simulink model "task1"  (R2023b)
settings: Solver=VariableStepAuto  StartTime=0.0  StopTime=100  RelTol=1e-3
settings Model: Creator=Notebook  LastModifiedBy=Notebook

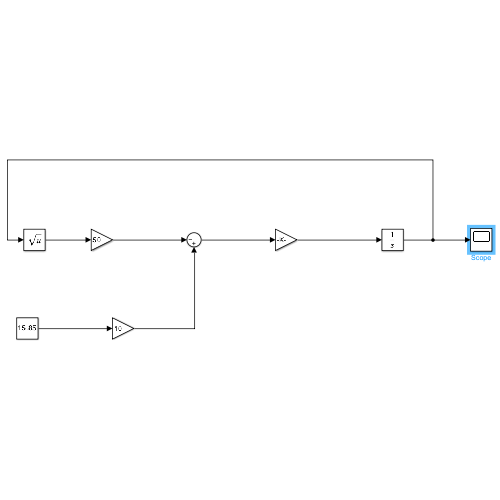
[thumbnail: Simulink's stored preview of the top-level diagram]
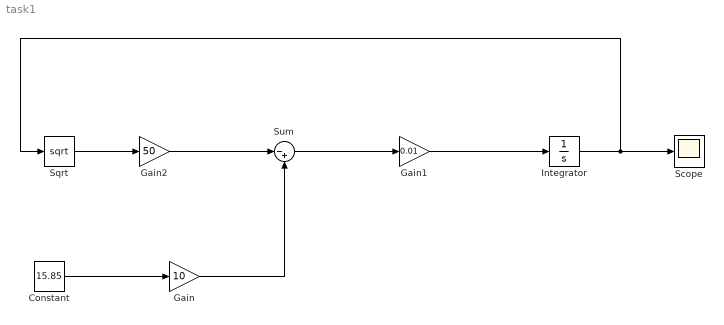
== system task1 ==
  Constant : Constant  Value=15.85
  Gain : Gain  Gain=10
  Gain1 : Gain  Gain=0.01
  Gain2 : Gain  Gain=50
  Integrator : Integrator  InitialCondition=2
  Scope : Scope
  Sqrt : Sqrt
  Sum : Sum  Inputs=|-+
  wires:
  Gain/1 -> Sum/2
  Constant/1 -> Gain/1
  Sqrt/1 -> Gain2/1
  Gain2/1 -> Sum/1
  Sum/1 -> Gain1/1
  Gain1/1 -> Integrator/1
  Integrator/1 -> Sqrt/1, Scope/1
